simulink model "dvopolozajni_relej"  (R2023a)
settings: Solver=ode45  StartTime=0.0  StopTime=tsim  MaxStep=1e-3  RelTol=1e-3  EnableMultiTasking=on
values from neighbouring files (symbols this model uses):
  a = 0.2    [simulacijska_provjera.m]
  C = 20    [simulacijska_provjera.m]
  x0 = 0    [simulacijska_provjera.m]
  y0 = 1    [simulacijska_provjera.m]
settings Model: Creator=Lea  LastModifiedBy=Enio
settings SolverCC: AlgebraicLoopSolver=TrustRegion
settings DataIOCC: LimitDataPoints=on  SaveFormat=Array  ReturnWorkspaceOutputs=off
settings OptimizationCC: LifeSpan=inf
settings DebuggingCC: UnconnectedInputMsg=warning  UnconnectedOutputMsg=warning  UnconnectedLineMsg=warning  SFUnexpectedBacktrackingDiag=warning  SFNoUnconditionalDefaultTransitionDiag=warning  SFExecutionAtInitializationDiag=none  ArithmeticOperatorsInVariantConditions=warning
settings HardwareCC: ProdBitPerPointer=32  ProdBitPerSizeT=32  ProdBitPerPtrDiffT=32  ProdLargestAtomicFloat=None  ProdIntDivRoundTo=Undefined  ProdEndianess=Unspecified  ProdWordSize=32  ProdHWDeviceType=32-bit Generic
settings ModelReferenceCC: EnableRefExpFcnMdlSchedulingChecks=on  PropagateSignalLabelsOutOfModel=off
settings SFSimCC: SimUseLocalCustomCode=off  CustomCodeUndefinedFunction=UseInterfaceOnly
settings RTWCC: RTWUseLocalCustomCode=off  DLArmComputeVersion=19.05
settings CodeAppCC: StateflowObjectComments=on
settings GRTTargetCC: TargetLangStandard=C89/C90 (ANSI)
settings ConfigComp: CovMetricSettings=dw  CovSaveCumulativeToWorkspaceVar=on  CovSaveSingleToWorkspaceVar=on  CovExternalEMLEnable=off

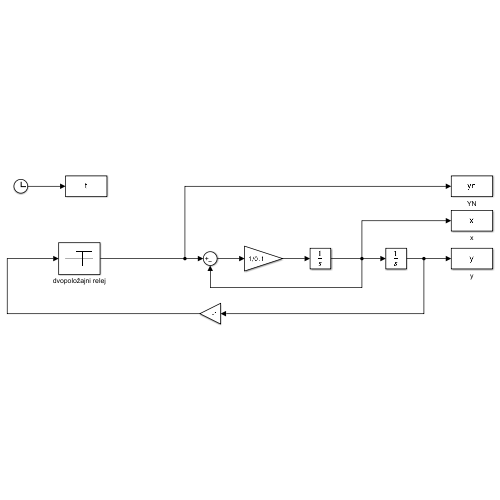
[thumbnail: Simulink's stored preview of the top-level diagram]
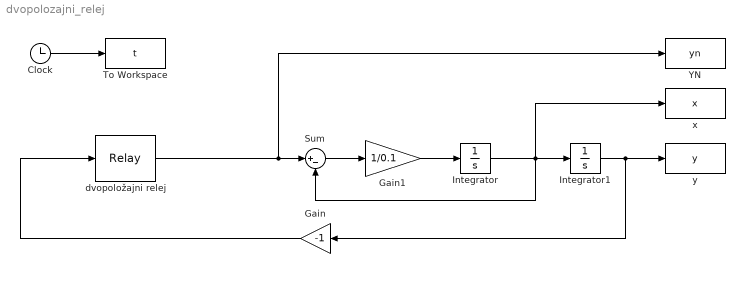
== system dvopolozajni_relej ==
  Clock : Clock
  Gain : Gain  Gain=-1
  Gain1 : Gain  Gain=1/0.1
  Integrator : Integrator  InitialCondition=x0
  Integrator1 : Integrator  InitialCondition=y0
  Sum : Sum  Inputs=|+-
  To Workspace : ToWorkspace  VariableName=t  SampleTime=-1
  YN : ToWorkspace  VariableName=yn  SampleTime=-1
  dvopoložajni relej : Relay  OnSwitchValue=a  OffSwitchValue=-a  OnOutputValue=C  OffOutputValue=-C
  x : ToWorkspace  VariableName=x  SampleTime=-1
  y : ToWorkspace  VariableName=y  SampleTime=-1
  wires:
  Gain1/1 -> Integrator/1
  Integrator/1 -> Integrator1/1, Sum/2, x/1
  Sum/1 -> Gain1/1
  Integrator1/1 -> Gain/1, y/1
  Clock/1 -> To Workspace/1
  Gain/1 -> dvopoložajni relej/1
  dvopoložajni relej/1 -> YN/1, Sum/1
